simulink model "Wishbone_loads"  (R2024b)
settings: Solver=VariableStepAuto  StartTime=0.0  StopTime=10.0  RelTol=1e-3
libraries: simulink x6
(part 2 of 2)

== system Wishbone_loads/Maximum acceleraton load cases for a front and rear wheel/Static front axle load(Wf) ==
  L : Inport
  L1 : Inport  Port=2
  In3 : Inport  Port=3
  W x (L-lm)/Lt : Product
  front wheel load bearing ratio (L-lm)/L : Subsystem
  Static front axle load(Wf) : Outport
  wires:
  W x (L-lm)/Lt/1 -> Static front axle load(Wf)/1  "Static front axle load(Wf)"
  front wheel load bearing ratio (L-lm)/L/1(Out1) -> W x (L-lm)/Lt/2  "front wheel load bearing ratio"
  L1/1 -> W x (L-lm)/Lt/1
  L/1 -> front wheel load bearing ratio (L-lm)/L/1(L)
  In3/1 -> front wheel load bearing ratio (L-lm)/L/2(In2)

== system Wishbone_loads/Maximum acceleraton load cases for a front and rear wheel/Static rear axle load(Wr) ==
  L : Inport
  L1 : Inport  Port=2
  In3 : Inport  Port=3
  W x lm/Lt : Product
  rear wheel load bearing ratio lm/L : Subsystem
  Static rear axle load(Wr) : Outport
  wires:
  W x lm/Lt/1 -> Static rear axle load(Wr)/1  "Static rear axle load(Wr)"
  rear wheel load bearing ratio lm/L/1(Out1) -> W x lm/Lt/2  "rear wheel load bearing ratio"
  L1/1 -> W x lm/Lt/1
  L/1 -> rear wheel load bearing ratio lm/L/1(In1)
  In3/1 -> rear wheel load bearing ratio lm/L/2(In2)

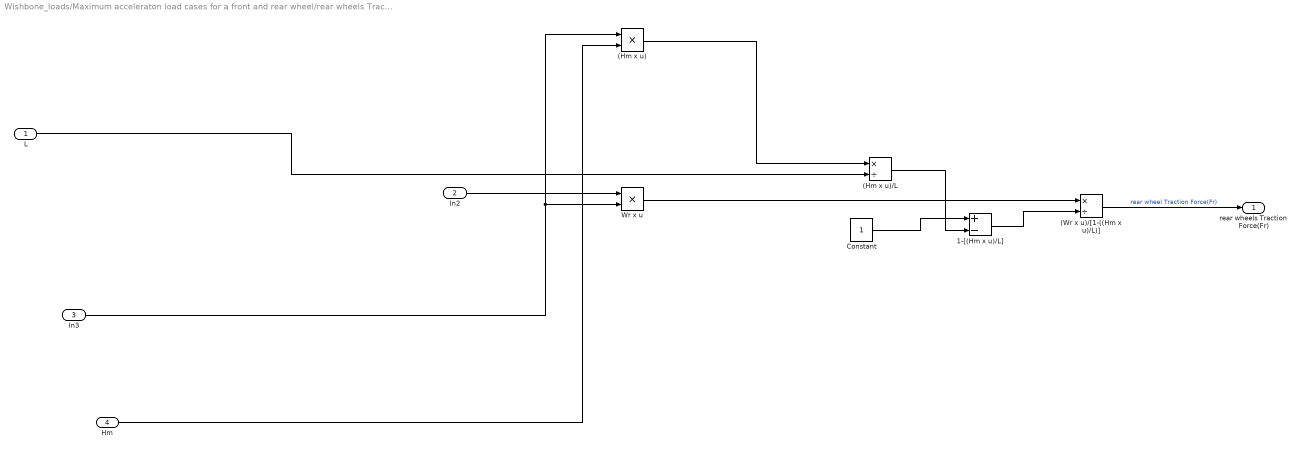
== system Wishbone_loads/Maximum acceleraton load cases for a front and rear wheel/rear wheels Traction Force(Fr) = (Wr x u)//[1-((Hm x u)//L)] ==
  L : Inport
  In2 : Inport  Port=2
  In3 : Inport  Port=3
  Hm : Inport  Port=4
  (Hm x u) : Product
  (Hm x u)/L : Product  Inputs=*/
  (Wr x u)/[1-((Hm x u)/L)] : Product  Inputs=*/
  1-[(Hm x u)/L] : Sum  Inputs=+-
  Constant : Constant
  Wr x u : Product
  rear wheels Traction Force(Fr) : Outport
  wires:
  In2/1 -> Wr x u/1
  In3/1 -> (Hm x u)/1, Wr x u/2
  (Hm x u)/1 -> (Hm x u)/L/1
  1-[(Hm x u)/L]/1 -> (Wr x u)/[1-((Hm x u)/L)]/2
  Wr x u/1 -> (Wr x u)/[1-((Hm x u)/L)]/1
  (Wr x u)/[1-((Hm x u)/L)]/1 -> rear wheels Traction Force(Fr)/1  "rear wheel Traction Force(Fr)"
  Hm/1 -> (Hm x u)/2
  L/1 -> (Hm x u)/L/2
  Constant/1 -> 1-[(Hm x u)/L]/1
  (Hm x u)/L/1 -> 1-[(Hm x u)/L]/2

== system Wishbone_loads/Maximum breaking load cases for a front and rear wheel/Effective Total weight of car ==
  In1 : Inport
  In2 : Inport  Port=2
  W+D : Sum
  Wx3.3 : Product
  effective total weight of car : Outport
  wires:
  W+D/1 -> effective total weight of car/1  "effective total weight of car"
  In2/1 -> W+D/1, Wx3.3/1
  Wx3.3/1 -> W+D/2  "max Downforce"
  In1/1 -> Wx3.3/2

== system Wishbone_loads/Maximum breaking load cases for a front and rear wheel/Front wheel vertical load (individual wheel) =(WF+deltaWx)//2 ==
  In1 : Inport
  Front Axle vertical load (WF) : Inport  Port=2
  (WF+deltaWx) : Sum
  (WF+deltaWx)/2 : Product
  Constant : Constant  Value=0.5
  Front wheel vertical load (individual wheel) : Outport
  wires:
  (WF+deltaWx)/1 -> (WF+deltaWx)/2/1  "Front wheel vertical loads"
  Constant/1 -> (WF+deltaWx)/2/2
  In1/1 -> (WF+deltaWx)/1
  (WF+deltaWx)/2/1 -> Front wheel vertical load (individual wheel)/1  "Front wheel vertical loads (individual wheel)"
  Front Axle vertical load (WF)/1 -> (WF+deltaWx)/2

== system Wishbone_loads/Maximum breaking load cases for a front and rear wheel/Longitudinal weight transfer (deltaWx)=(FxHm)//L ==
  L : Inport
  Hm : Inport  Port=2
  In2 : Inport  Port=3
  (FxHm) : Product
  (FxHm)/L : Product  Inputs=*/
  Longitudinal weight transfer (deltaWx) : Outport
  wires:
  (FxHm)/1 -> (FxHm)/L/1  "(FxHm)"
  Hm/1 -> (FxHm)/1
  L/1 -> (FxHm)/L/2
  In2/1 -> (FxHm)/2
  (FxHm)/L/1 -> Longitudinal weight transfer (deltaWx)/1  "Longitudinal weight transfer (deltaWx)"

== system Wishbone_loads/Maximum breaking load cases for a front and rear wheel/Rear wheel vertical load (individual wheel) =(WR-deltaWx)//2 ==
  Longitudinal weight transfer (deltaWx) : Inport
  Rear Axle vertical load (WF) : Inport  Port=2
  (WF+deltaWx) : Sum  Inputs=-+
  (WF+deltaWx)/2 : Product
  Constant : Constant  Value=0.5
  Rear wheel vertical load (individual wheel) : Outport
  wires:
  (WF+deltaWx)/1 -> (WF+deltaWx)/2/1  "Front wheel vertical loads"
  Constant/1 -> (WF+deltaWx)/2/2
  Longitudinal weight transfer (deltaWx)/1 -> (WF+deltaWx)/1
  (WF+deltaWx)/2/1 -> Rear wheel vertical load (individual wheel)/1  "Front wheel vertical loads (individual wheel)"
  Rear Axle vertical load (WF)/1 -> (WF+deltaWx)/2

== system Wishbone_loads/Maximum breaking load cases for a front and rear wheel/front wheel load bearing ratio (L-lm)//L ==
  In1 : Inport
  In2 : Inport  Port=2
  (L-lm)/L : Product  Inputs=*/
  L-lm : Sum  Inputs=+-
  Out1 : Outport
  wires:
  In1/1 -> (L-lm)/L/2, L-lm/1
  L-lm/1 -> (L-lm)/L/1
  In2/1 -> L-lm/2
  (L-lm)/L/1 -> Out1/1

== system Wishbone_loads/Maximum breaking load cases for a front and rear wheel/rear wheel load bearing ratio lm//L ==
  In1 : Inport
  In2 : Inport  Port=2
  Divide : Product  Inputs=*/
  Out1 : Outport
  wires:
  In1/1 -> Divide/2
  Divide/1 -> Out1/1
  In2/1 -> Divide/1

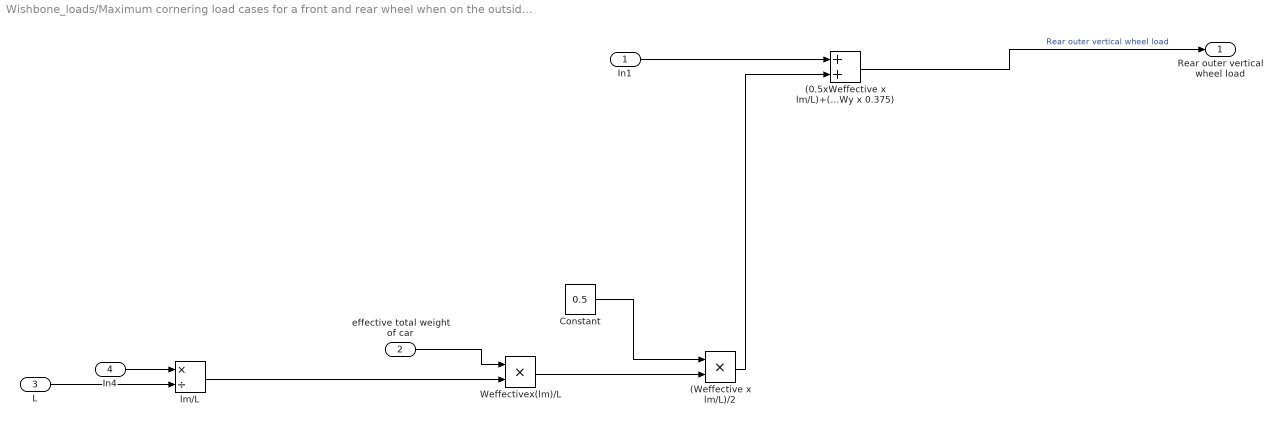
== system Wishbone_loads/Maximum cornering load cases for a front and rear wheel when on the outside of a corner/(0.5xWeffective x lm//L)+(deltaWy x 0.375) ==
  In1 : Inport
  effective total weight of car : Inport  Port=2
  L : Inport  Port=3
  In4 : Inport  Port=4
  (0.5xWeffective x lm/L)+(deltaWy x 0.375) : Sum
  (Weffective x lm/L)/2 : Product
  Constant : Constant  Value=0.5
  Weffectivex(lm)/L : Product
  lm/L : Product  Inputs=*/
  Rear outer vertical wheel load : Outport
  wires:
  Weffectivex(lm)/L/1 -> (Weffective x lm/L)/2/2
  In1/1 -> (0.5xWeffective x lm/L)+(deltaWy x 0.375)/1
  (Weffective x lm/L)/2/1 -> (0.5xWeffective x lm/L)+(deltaWy x 0.375)/2
  Constant/1 -> (Weffective x lm/L)/2/1
  (0.5xWeffective x lm/L)+(deltaWy x 0.375)/1 -> Rear outer vertical wheel load/1  "Rear outer vertical wheel load"
  lm/L/1 -> Weffectivex(lm)/L/2
  L/1 -> lm/L/2
  In4/1 -> lm/L/1
  effective total weight of car/1 -> Weffectivex(lm)/L/1

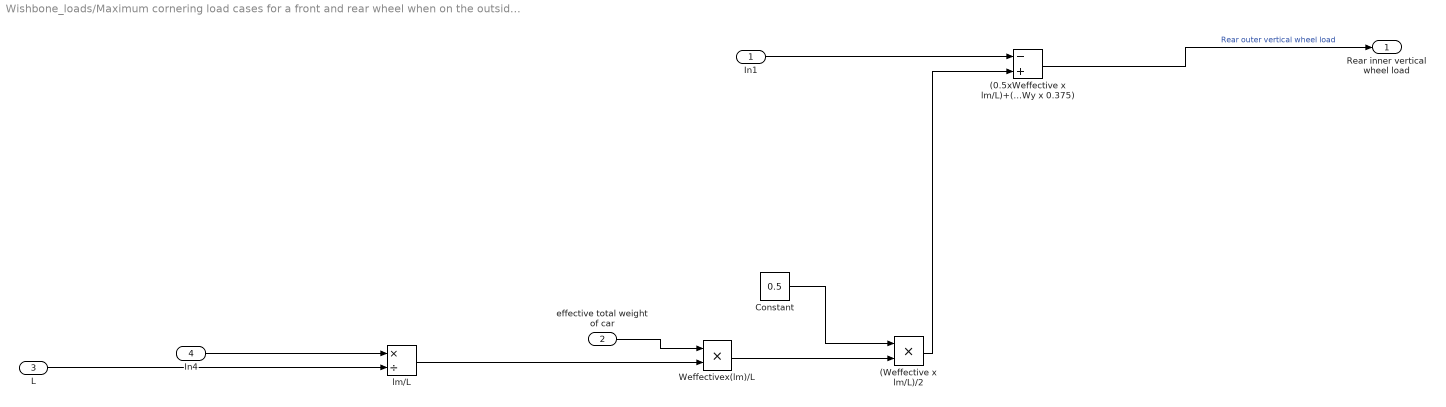
== system Wishbone_loads/Maximum cornering load cases for a front and rear wheel when on the outside of a corner/(0.5xWeffective x lm//L)-(deltaWy x 0.375)1 ==
  In1 : Inport
  effective total weight of car : Inport  Port=2
  L : Inport  Port=3
  In4 : Inport  Port=4
  (0.5xWeffective x lm/L)+(deltaWy x 0.375) : Sum  Inputs=-+
  (Weffective x lm/L)/2 : Product
  Constant : Constant  Value=0.5
  Weffectivex(lm)/L : Product
  lm/L : Product  Inputs=*/
  Rear inner vertical wheel load : Outport
  wires:
  Weffectivex(lm)/L/1 -> (Weffective x lm/L)/2/2
  In1/1 -> (0.5xWeffective x lm/L)+(deltaWy x 0.375)/1
  (Weffective x lm/L)/2/1 -> (0.5xWeffective x lm/L)+(deltaWy x 0.375)/2
  Constant/1 -> (Weffective x lm/L)/2/1
  (0.5xWeffective x lm/L)+(deltaWy x 0.375)/1 -> Rear inner vertical wheel load/1  "Rear outer vertical wheel load"
  lm/L/1 -> Weffectivex(lm)/L/2
  L/1 -> lm/L/2
  In4/1 -> lm/L/1
  effective total weight of car/1 -> Weffectivex(lm)/L/1

== system Wishbone_loads/Maximum cornering load cases for a front and rear wheel when on the outside of a corner/Effective Total weight of car ==
  In1 : Inport
  In2 : Inport  Port=2
  W+D : Sum
  Wx3.3 : Product
  effective total weight of car : Outport
  wires:
  W+D/1 -> effective total weight of car/1  "effective total weight of car"
  In2/1 -> W+D/1, Wx3.3/1
  Wx3.3/1 -> W+D/2  "max Downforce"
  In1/1 -> Wx3.3/2

== system Wishbone_loads/Maximum cornering load cases for a front and rear wheel when on the outside of a corner/Lateral weight transfer (deltaWy)=(FxHm)//T ==
  Hm : Inport
  In2 : Inport  Port=2
  T : Inport  Port=3
  (FxHm) : Product
  (FxHm)/T : Product  Inputs=*/
  Lateral weight transfer (deltaWy) : Outport
  wires:
  (FxHm)/1 -> (FxHm)/T/1  "(FxHm)"
  Hm/1 -> (FxHm)/1
  T/1 -> (FxHm)/T/2
  In2/1 -> (FxHm)/2
  (FxHm)/T/1 -> Lateral weight transfer (deltaWy)/1  "Lateral weight transfer (deltaWy)"

== system Wishbone_loads/Maximum cornering load cases for a front and rear wheel when on the outside of a corner/effective weight of one front wheel ==
  In1 : Inport
  front wheel load bearing ratio (L-lm)/L : Inport  Port=2
  (Weffectivex(L-lm)/L)/2 : Product
  Constant : Constant  Value=0.5
  Weffectivex(L-lm)/L : Product
  effective weight of one front wheel : Outport
  wires:
  Constant/1 -> (Weffectivex(L-lm)/L)/2/1
  (Weffectivex(L-lm)/L)/2/1 -> effective weight of one front wheel/1
  Weffectivex(L-lm)/L/1 -> (Weffectivex(L-lm)/L)/2/2
  In1/1 -> Weffectivex(L-lm)/L/2
  front wheel load bearing ratio (L-lm)/L/1 -> Weffectivex(L-lm)/L/1

== system Wishbone_loads/Maximum cornering load cases for a front and rear wheel when on the outside of a corner/front wheel load bearing ratio (L-lm)//L ==
  In1 : Inport
  In2 : Inport  Port=2
  (L-lm)/L : Product  Inputs=*/
  L-lm : Sum  Inputs=+-
  Out1 : Outport
  wires:
  In1/1 -> (L-lm)/L/2, L-lm/1
  L-lm/1 -> (L-lm)/L/1
  In2/1 -> L-lm/2
  (L-lm)/L/1 -> Out1/1

== system Wishbone_loads/Maximum vertical load cases for a front and rear wheels/design vertical load for one front wheel ==
  In1 : Inport
  In2 : Inport  Port=2
  " design vertical load per side x (L-lm)/L" : Product
  Design Vertical load of one front wheel : Outport
  wires:
  " design vertical load per side x (L-lm)/L"/1 -> Design Vertical load of one front wheel/1  "Design Vertical load of one front wheel"
  In2/1 -> " design vertical load per side x (L-lm)/L"/2
  In1/1 -> " design vertical load per side x (L-lm)/L"/1

== system Wishbone_loads/Maximum vertical load cases for a front and rear wheels/design vertical load for one rear wheel ==
  In1 : Inport
  In2 : Inport  Port=2
  "design vertical load per side x lm/L  " : Product
  Design Vertical load of one rear wheel : Outport
  wires:
  In2/1 -> "design vertical load per side x lm/L  "/2
  In1/1 -> "design vertical load per side x lm/L  "/1
  "design vertical load per side x lm/L  "/1 -> Design Vertical load of one rear wheel/1  "Design Vertical load of one raer wheel"

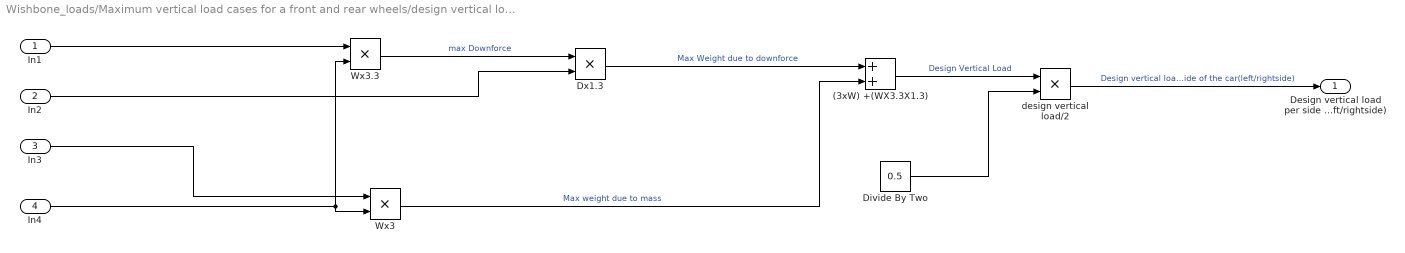
== system Wishbone_loads/Maximum vertical load cases for a front and rear wheels/design vertical load per side of the car (eg left//right side) ==
  In1 : Inport
  In2 : Inport  Port=2
  In3 : Inport  Port=3
  In4 : Inport  Port=4
  (3xW) +(WX3.3X1.3) : Sum
  Divide By Two : Constant  Value=0.5
  Dx1.3 : Product
  Wx3 : Product
  Wx3.3 : Product
  design vertical load/2 : Product
  Design vertical load per side of the car(left/rightside) : Outport
  wires:
  In4/1 -> Wx3/2, Wx3.3/2
  In1/1 -> Wx3.3/1
  (3xW) +(WX3.3X1.3)/1 -> design vertical load/2/1  "Design Vertical Load"
  design vertical load/2/1 -> Design vertical load per side of the car(left/rightside)/1  "Design vertical load per side of the car(left/rightside)"
  Wx3.3/1 -> Dx1.3/1  "max Downforce"
  Dx1.3/1 -> (3xW) +(WX3.3X1.3)/1  "Max Weight due to downforce"
  Wx3/1 -> (3xW) +(WX3.3X1.3)/2  "Max weight due to mass"
  Divide By Two/1 -> design vertical load/2/2
  In2/1 -> Dx1.3/2
  In3/1 -> Wx3/1

== system Wishbone_loads/Maximum vertical load cases for a front and rear wheels/front wheel load bearing ratio (L-lm)//L ==
  In1 : Inport
  In2 : Inport  Port=2
  (L-lm)/L : Product  Inputs=*/
  L-lm : Sum  Inputs=+-
  Out1 : Outport
  wires:
  In1/1 -> (L-lm)/L/2, L-lm/1
  L-lm/1 -> (L-lm)/L/1
  In2/1 -> L-lm/2
  (L-lm)/L/1 -> Out1/1

== system Wishbone_loads/Maximum vertical load cases for a front and rear wheels/rear wheel load bearing ratio lm//L ==
  In1 : Inport
  In2 : Inport  Port=2
  Divide : Product  Inputs=*/
  Out1 : Outport
  wires:
  In1/1 -> Divide/2
  Divide/1 -> Out1/1
  In2/1 -> Divide/1

== system Wishbone_loads/Maximum acceleraton load cases for a front and rear wheel/Front wheel loads(Wfl and Wfr)=(Wr- deltaWx)//2/Longitudinal weight transfer (deltaWx)=(FrxHm)//L ==
  Hm : Inport
  Traction Force(Fr) : Inport  Port=2
  L : Inport  Port=3
  (FxHm) : Product
  (FxHm)/L : Product  Inputs=*/
  Longitudinal weight transfer (deltaWx) : Outport
  wires:
  (FxHm)/1 -> (FxHm)/L/1  "(FxHm)"
  Hm/1 -> (FxHm)/1
  L/1 -> (FxHm)/L/2
  Traction Force(Fr)/1 -> (FxHm)/2
  (FxHm)/L/1 -> Longitudinal weight transfer (deltaWx)/1  "Longitudinal weight transfer (deltaWx)"

== system Wishbone_loads/Maximum acceleraton load cases for a front and rear wheel/Rear wheel loads(Wrl and Wrr)=(Wr+ deltaWx)//2/Longitudinal weight transfer (deltaWx)=(FxHm)//L ==
  Hm : Inport
  Traction Force(F) : Inport  Port=2
  L : Inport  Port=3
  (FxHm) : Product
  (FxHm)/L : Product  Inputs=*/
  Longitudinal weight transfer (deltaWx) : Outport
  wires:
  (FxHm)/1 -> (FxHm)/L/1  "(FxHm)"
  Hm/1 -> (FxHm)/1
  L/1 -> (FxHm)/L/2
  Traction Force(F)/1 -> (FxHm)/2
  (FxHm)/L/1 -> Longitudinal weight transfer (deltaWx)/1  "Longitudinal weight transfer (deltaWx)"

== system Wishbone_loads/Maximum acceleraton load cases for a front and rear wheel/Static front axle load(Wf)/front wheel load bearing ratio (L-lm)//L ==
  L : Inport
  In2 : Inport  Port=2
  (L-lm)/L : Product  Inputs=*/
  L-lm : Sum  Inputs=+-
  Out1 : Outport
  wires:
  L/1 -> (L-lm)/L/2, L-lm/1
  L-lm/1 -> (L-lm)/L/1
  In2/1 -> L-lm/2
  (L-lm)/L/1 -> Out1/1

== system Wishbone_loads/Maximum acceleraton load cases for a front and rear wheel/Static rear axle load(Wr)/rear wheel load bearing ratio lm//L ==
  In1 : Inport
  In2 : Inport  Port=2
  Divide : Product  Inputs=*/
  Out1 : Outport
  wires:
  In1/1 -> Divide/2
  Divide/1 -> Out1/1
  In2/1 -> Divide/1
